simulink model "MotorSpeedController"  (R2016b)
settings: Solver=FixedStepAuto  StartTime=0.0  StopTime=10.0  RelTol=1e-3
PreLoadFcn:
  | waijung.modelPreload; % Required for working with Waijung Blockset. Do not remove.
InitFcn:
  | cubeparameters
undefined symbols (not defined in the file): K, Link, LQFP100, ST, STM32F407VG, STM32F4DISCOVERY, Ts
libraries: stm32f4_io_lib x3, simulink x1, stm32f4_adc_lib x1, stm32f4_device_config_lib x1, BC_USB x1
CloseFcn:
  | waijung.modelClose; % Required for working with Waijung Blockset. Do not remove.
settings Model: Creator=Wall  LastModifiedBy=Wall
settings OptimizationCC: DefaultParameterBehavior=Inlined
settings DebuggingCC: ParameterTunabilityLossMsg=error
settings HardwareCC: ProdBitPerPointer=32  ProdBitPerSizeT=32  ProdBitPerPtrDiffT=32  ProdLargestAtomicFloat=None  ProdIntDivRoundTo=Undefined  ProdWordSize=32  ProdHWDeviceType=ARM Compatible->Cortex - M4  TargetEndianess=LittleEndian  TargetHWDeviceType=ARM Compatible->Cortex - M4
settings RTWCC: SystemTargetFile=stm32f4.tlc  GenerateMakefile=off  TemplateMakefile=ert_default_tmf  Description=STM32F4 Target  GenerateReport=on  IncludeHyperlinkInReport=on  GenerateTraceInfo=on  GenerateTraceReport=on  GenerateTraceReportSl=on  GenerateTraceReportSf=on  GenerateTraceReportEml=on
settings CodeAppCC: ForceParamTrailComments=on  IgnoreCustomStorageClasses=off  OperatorAnnotations=on  SimulinkDataObjDesc=on  SFDataObjDesc=on  MATLABFcnDesc=on  InsertBlockDesc=on  MATLABSourceComments=on
settings STFCustomTargetCC: TargetLangStandard=C99 (ISO)  ModelReferenceCompliant=off  CombineOutputUpdateFcns=on  ERTCustomFileBanners=on  SupportContinuousTime=off  SupportNonInlinedSFcns=off  RemoveResetFunc=on  MATLABClassNameForMDSCustomization=Simulink.SoftwareTarget.ERTCustomization  GRTInterface=off  SystemTargetFile=stm32f4.tlc
settings ERTTargetCC: TargetLangStandard=C99 (ISO)  ModelReferenceCompliant=off  ParMdlRefBuildCompliant=off  CompOptLevelCompliant=off  ConcurrentExecutionCompliant=off  ERTFirstTimeCompliant=off  ModelStepFunctionPrototypeControlCompliant=off  CPPClassGenCompliant=off  UseToolchainInfoCompliant=off  InlinedParameterPlacement=NonHierarchical  ERTSrcFileBannerTemplate=stm32f4_code_template.cgt  ERTHdrFileBannerTemplate=stm32f4_code_template.cgt  ERTDataSrcFileTemplate=stm32f4_code_template.cgt  ERTDataHdrFileTemplate=stm32f4_code_template.cgt  ERTCustomFileTemplate=stm32f4_file_process.tlc

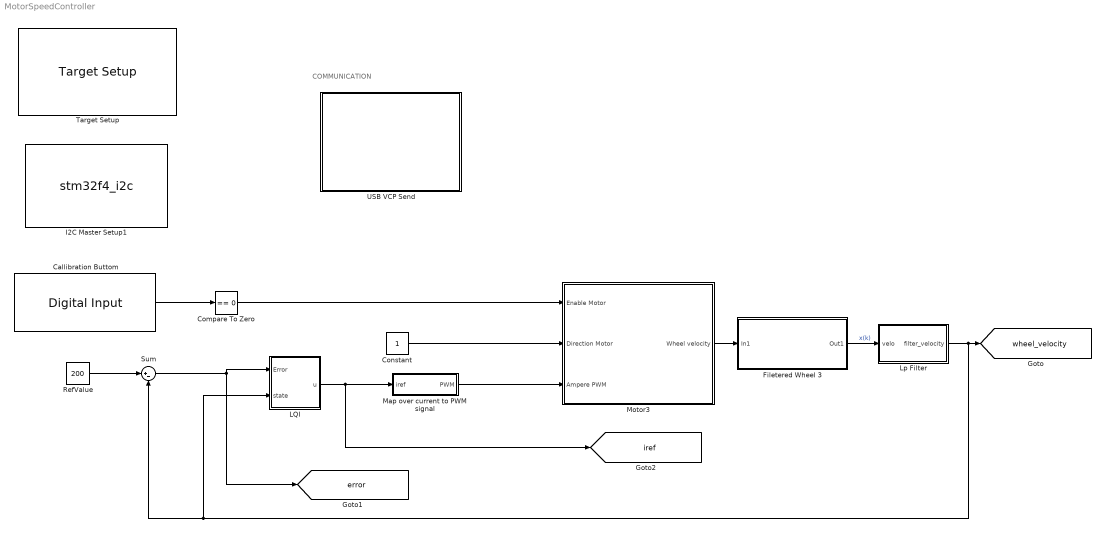
== system MotorSpeedController ==
  note: COMMUNICATION
  Callibration Buttom : stm32f4_io_lib/Digital Input  port=E  speed=100  porttype=Pull Up  porttypestr=UP  use_pin0=off  use_pin1=off  use_pin2=off  use_pin3=off  use_pin4=off  use_pin5=off  use_pin6=off  use_pin7=off  use_pin8=off  use_pin9=off  use_pin10=on  use_pin11=off  use_pin12=off  use_pin13=off  use_pin14=off  use_pin15=off  pinstr=GPIO_Pin_10  usedpinarray="[0  0  0  0  0  0  0  0  0  0  1  0  0  0  0  0]"  bitbandingstr="#define CallibrationButtom_E10 Peripheral_BB(GPIOE->IDR, 10)  /* Output pin */"  sampletime=Ts.controller  sampletimestr=0.016  blockid=CallibrationButtom  enablecustomportlabel=off  glabalinit=off  cinputportlabel=In1, In2  coutputportlabel=Out1, Out2
  Compare To Zero : simulink/Logic and Bit Operations/Compare To Zero  relop===  OutDataTypeStr=boolean
  Constant : Constant  SampleTime=Ts.controller
  Filetered Wheel 3 : Subsystem
  I2C Master Setup1 : S-Function  FunctionName=stm32f4_i2c  Parameters=configuration,module,transfer,clkspeed,timeout,sdapin,sclpin,writecount,readcount,inputtypearray,outputtypearray,confstr,sampletime,sampletimestr,blockid  SFunctionDeploymentMode=off  EnableBusSupport=off  mask(stm32f4_i2c){configuration=Setup, module=1, lastmodule=1, transfer=Blocking, dutycycle=TLow/THigh = 2, clkspeed=400, timeout=25, writecount=0, readcount=0, sdapin=B9, sclpin=B6, waitwritetime=0, inputtypearray=[0], outputtypearray=[0], confstr=["B","9","B","6","1","1","6","0","I2C_DutyCycle_2","0","off"], sampletime=-1, sampletimestr=0.002, blockid=I2CMasterSetup1}
      mask prompts: module "I2C Module"; lastmodule "Last module"; transfer "Transfer mode"; dutycycle "Duty cycle in fast mode"; clkspeed "Clock speed (kHz)"; timeout "Timeout (ms)"; writecount "Bytes write count"; readcount "Bytes read count"; sdapin "SDA pin"; sclpin "SCL pin"; waitwritetime "Wait write time (ms), default is 0"; inputtypearray "Input type array"; outputtypearray "Output type array"; confstr "Configuration string"; sampletime "Sample time (sec)"; sampletimestr "Compiled sample time (sec) in string"
      mask init:
      | stm32f4_i2c_callback('init');
      mask Help: web(fullfile(waijungdocroot,'stm32f4_i2c_setup.htm'), '-browser')
      mask TypeOptions configuration: Setup | Transaction
      mask Callback configuration: stm32f4_i2c_callback('configuration');
      mask TypeOptions module: 1 | 2 | 3
      mask Callback module: stm32f4_i2c_callback('module');
      mask TypeOptions transfer: Blocking | Non-blocking
      mask TypeOptions dutycycle: TLow/THigh = 16/9 | TLow/THigh = 2
      mask Callback dutycycle: stm32f4_i2c_callback('dutycycle');
      mask Callback writecount: stm32f4_i2c_callback('writecount');
      mask Callback readcount: stm32f4_i2c_callback('readcount');
      mask TypeOptions sdapin: - | B7 | B9
      mask Callback sdapin: stm32f4_i2c_callback('sdapin');
      mask TypeOptions sclpin: - | B6 | B8
      mask Callback sclpin: stm32f4_i2c_callback('sclpin');
      mask Callback confstr: stm32f4_i2c_callback('confstr');
      mask Callback sampletime: stm32f4_i2c_callback('sampletime');
      mask Callback sampletimestr: stm32f4_i2c_callback('sampletimestr');
      mask Callback blockid: stm32f4_i2c_callback('blockid');
      mask Display: text(0.5, 0.5, 'Module: I2C1\nClock: 400kHz\nSDA/SCL Pin: B9/B6','ver','middle','hor','center');
  LQI : Subsystem
  Lp Filter : MATLAB Function  TreatAsAtomicUnit=on
  Map over current to PWM signal : Subsystem
  Motor3 : Subsystem
  RefValue : Constant  Value=200  SampleTime=Ts.controller
  Sum : Sum  Inputs=|+-
  Target Setup : stm32f4_device_config_lib/Target Setup  Priority=100  compiler=GNU ARM  previous_compiler=GNU ARM  mcu=STM32F407VG (LQFP100); STM32F4DISCOVERY  mcustr=STM32F407VG  clockconfig=STM32F4DISCOVERY Default (HSEOSC-8MHz/HCLK-168MHz)  system_stm32f4xx_c_path=C:\waijung15_04a\targets\stm32f4_target\stm32f4\utils\STM32F4xx_AN3988_V1.0.1\stm32f4_default\hseosc8mhz  showmemoryconfiguration=off  stacksize=0x400  heapsize=0x200  enableautocompiledownload=on  fullchiperase=off  programmerinterface=ST-Link  editctrlstr=on  compilercontrolstr=$(patsubst %, -I%, .) -mcpu=cortex-m4 -mthumb -mthumb-interwork -mfloat-abi=hard -mfpu=fpv4-sp-d16 -ffast-math -Wall -Wextra -Ofast  assemblercontrolstr=$(patsubst %, -I%, .) -mcpu=cortex-m4 -mthumb -mthumb-interwork -mfloat-abi=hard -mfpu=fpv4-sp-d16 -ffast-math -Wall -Wextra -Ofast -Wa,-amhls=$(<:.s=.lst) -D__STACK_SIZE=$(STACK_SIZE) -D__HEAP_SIZE=$(HEAP_SIZE)  linkercontrolstr=-T$(LD_SCRIPT) -g -Wl,-Map=$(MAP),--cref,--no-warn-mismatch -mcpu=cortex-m4 -mthumb -mthumb-interwork -mfloat-abi=hard -mfpu=fpv4-sp-d16  runafterdownload=on  execprofile=None  profileruart=1  profilerbaud=115200  profilertxpin=Not used  profilerinitstr=0.002,168000000,336000,115200,0  manualsetsampletime=on  sampletime=0.002  blockid=TargetSetup  systickreloadvalue=336000  hseval=8000000  lastprofileruart=1  hclk=168000000  flashorigin=0x8000000  flashlength=1M  ramorigin=0x20000000  ramlength=112k  useextram=off
  USB VCP Send : Subsystem
  tag scope: error=global, iref=global, wheel_velocity=global
  wires:
  Callibration Buttom/1 -> Compare To Zero/1
  Constant/1 -> Motor3/2("Direction Motor ")
  Motor3/1(Wheel velocity) -> Filetered Wheel 3/1(In1)
  Filetered Wheel 3/1(Out1) -> Lp Filter/1(velo)  "x(k)"
  RefValue/1 -> Sum/1
  Sum/1 -> [error], LQI/1(Error)
  LQI/1(u) -> [iref], Map over current to PWM signal/1(iref)
  Compare To Zero/1 -> Motor3/1(Enable Motor)
  Map over current to PWM signal/1(PWM) -> Motor3/3(Ampere PWM)
  Lp Filter/1(filter_velocity) -> LQI/2(state), Sum/2, [wheel_velocity]

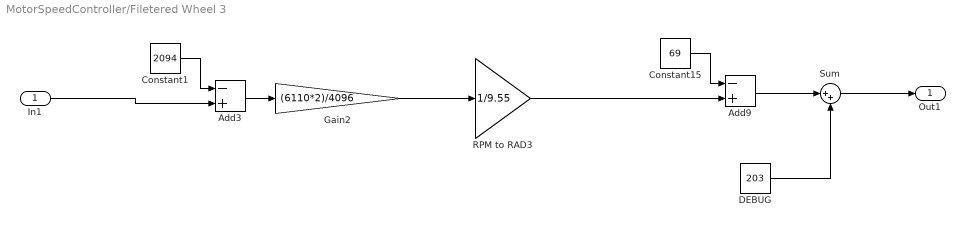
== system MotorSpeedController/Filetered Wheel 3 ==
  In1 : Inport
  Add3 : Sum  Inputs=-+
  Add9 : Sum  Inputs=-+
  Constant1 : Constant  Value=2094  SampleTime=Ts.controller
  Constant15 : Constant  Value=69  SampleTime=Ts.controller
  DEBUG : Constant  Value=203  SampleTime=Ts.controller
  Gain2 : Gain  Gain=(6110*2)/4096
  RPM to RAD3 : Gain  Gain=1/9.55
  Sum : Sum  Inputs=|++
  Out1 : Outport
  wires:
  Gain2/1 -> RPM to RAD3/1
  Add3/1 -> Gain2/1
  Constant1/1 -> Add3/1
  In1/1 -> Add3/2
  Constant15/1 -> Add9/1
  RPM to RAD3/1 -> Add9/2
  Add9/1 -> Sum/1
  Sum/1 -> Out1/1
  DEBUG/1 -> Sum/2

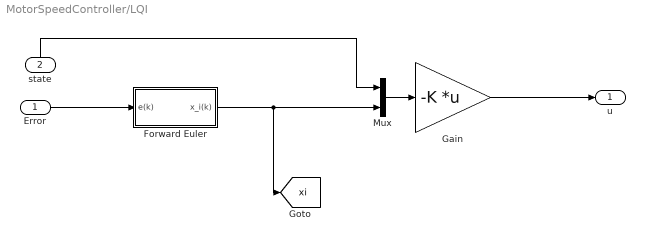
== system MotorSpeedController/LQI ==
  Error : Inport
  state : Inport  Port=2
  Forward Euler : Subsystem
  Gain : Gain  Gain=-K  Multiplication=Matrix(K*u) (u vector)
  Mux : Mux  Inputs=2
  u : Outport
  tag scope: xi=global
  wires:
  Forward Euler/1(x_i(k)) -> [xi], Mux/2
  Mux/1 -> Gain/1
  Error/1 -> Forward Euler/1(e(k))
  state/1 -> Mux/1
  Gain/1 -> u/1

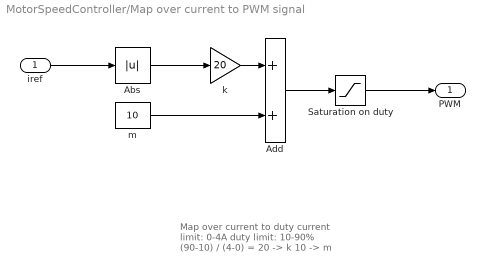
== system MotorSpeedController/Map over current to PWM signal ==
  note: Map over current to duty
      | current limit: 0-4A
      | duty limit: 10-90%
      |
      | (90-10) / (4-0) = 20 -> k
      | 10 -> m
  iref : Inport
  Abs : Abs
  Add : Sum
  Saturation on duty : Saturate  UpperLimit=90  LowerLimit=10  OutDataTypeStr=single
  k : Gain  Gain=20
  m : Constant  Value=10  OutDataTypeStr=single  SampleTime=Ts.controller
  PWM : Outport
  wires:
  Add/1 -> Saturation on duty/1
  Saturation on duty/1 -> PWM/1
  iref/1 -> Abs/1
  Abs/1 -> k/1
  k/1 -> Add/1
  m/1 -> Add/2

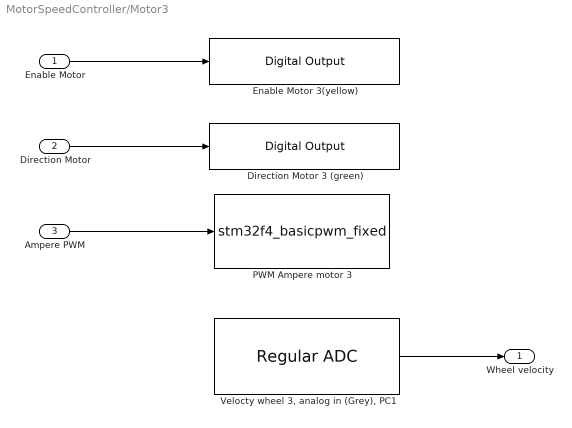
== system MotorSpeedController/Motor3 ==
  Enable Motor : Inport
  "Direction Motor " : Inport  Port=2
  Ampere PWM : Inport  Port=3
  Direction Motor 3 (green) : stm32f4_io_lib/Digital Output  use_bitband=on  port=D  speed=100  porttype=Push Pull  porttypestr=PP  use_pin0=off  use_pin1=off  use_pin2=off  use_pin3=off  use_pin4=off  use_pin5=off  use_pin6=off  use_pin7=off  use_pin8=off  use_pin9=off  use_pin10=off  use_pin11=on  use_pin12=off  use_pin13=off  use_pin14=off  use_pin15=off  pinstr=GPIO_Pin_11  usedpinarray="[0  0  0  0  0  0  0  0  0  0  0  1  0  0  0  0]"  bitbandingstr="#define Motor3DirectionMotor3green_D11 Peripheral_BB(GPIOD->ODR, 11)  /* Output pin */"  sampletime=-1  sampletimestr=0.016  blockid=Motor3DirectionMotor3green  enablecustomportlabel=off  globalinit=off  cinputportlabel=In1, In2  coutputportlabel=0
  Enable Motor 3(yellow) : stm32f4_io_lib/Digital Output  use_bitband=on  port=D  speed=100  porttype=Push Pull  porttypestr=PP  use_pin0=off  use_pin1=off  use_pin2=off  use_pin3=off  use_pin4=off  use_pin5=off  use_pin6=off  use_pin7=off  use_pin8=off  use_pin9=on  use_pin10=off  use_pin11=off  use_pin12=off  use_pin13=off  use_pin14=off  use_pin15=off  pinstr=GPIO_Pin_9  usedpinarray="[0  0  0  0  0  0  0  0  0  1  0  0  0  0  0  0]"  bitbandingstr="#define Motor3EnableMotor3yellow_D9 Peripheral_BB(GPIOD->ODR, 9)  /* Output pin */"  sampletime=-1  sampletimestr=0.016  blockid=Motor3EnableMotor3yellow  enablecustomportlabel=off  globalinit=off  cinputportlabel=In1, In2  coutputportlabel=0
  PWM Ampere motor 3 : S-Function  FunctionName=stm32f4_basicpwm_fixed  Parameters=timer,pwmperiod,uc3m_pwmperiod,ch1pin,ch2pin,ch3pin,ch4pin,sampletime,sampletimestr,blockid,apb,portstr,pinstr,pinmat,timarr,timprescale,chmat,polaritystr  SFunctionDeploymentMode=off  EnableBusSupport=off  mask(stm32f4_basicpwm_fixed){timer=2, pwmperiod=0.02, uc3m_pwmperiod=0.0002, polarity=Active High, polaritystr=TIM_OCPolarity_High, ch1pin=Not available - Do not use, ch2pin=Not available - Do not use, ch3pin=Not available - Do not use, ch4pin=A3, sampletime=-1, sampletimestr=0.016, blockid=Motor3PWMAmperemotor3, portpinstr=,,,A3, enablecustomportlabel=off, cinputportlabel=In1, In2, In3, In4, coutputportlabel=0, callbackgensrccode=off, apb=1, portstr=["A"], pinstr=["GPIO_Pin_3"], pinmat=[1 3], timarr=59999, timprescale=55, chmat=[4]}
      mask prompts: pwmperiod "PWM Period (seconds)"; uc3m_pwmperiod "PWM Signal Period (seconds)"; ch1pin "Channel 1"; ch2pin "Channel 2"; ch3pin "Channel 3"; ch4pin "Channel 4"; sampletime "Sample time (sec)"; sampletimestr "Compiled sample time (sec) in string"; portpinstr "Port pin string"; enablecustomportlabel "Enable custom port labels"; cinputportlabel "Custom input port labels (Ex. In1, In2, In3)"; coutputportlabel "Custom output port labels (Ex. Out1, Out2, Out3)"; callbackgensrccode "Gen source code from callback"; portstr "Port string"; pinstr "Pin string"; pinmat "Pin matrix"; timarr "Timer ARR"; timprescale "Timer PRESCALE"; chmat "Channel order"
      mask help:
      | This block implements basic Edge-aligned Pulse Width Modulation (PWM) generation.
      | All timers are 16-bit. The PWM period is fixed (per timer).
      |
      | This block was fixed by Sr Antonio
      mask init:
      | stm32f4_basicpwm_callback_fixed('init');
      mask Help: web(fullfile(waijungdocroot,'stm32f4_basicpwm.htm'),'-browser')
      mask TypeOptions timer: 1 | 2 | 3 | 4 | 5 | 8 | 9 | 10 | 11 | 12 | 13 | 14
      mask Callback timer: stm32f4_basicpwm_callback_fixed('timer');
      mask Callback pwmperiod: stm32f4_basicpwm_callback_fixed('pwmperiod');
      mask Callback uc3m_pwmperiod: stm32f4_basicpwm_callback_fixed('uc3m_pwmperiod');
      mask TypeOptions polarity: Active High | Active Low
      mask Callback polarity: stm32f4_basicpwm_callback_fixed('polarity');
      mask TypeOptions ch1pin: Not available - Do not use | A0 | A5
      mask Callback ch1pin: stm32f4_basicpwm_callback_fixed('ch1pin');
      mask TypeOptions ch2pin: Not available - Do not use | A1 | B3
      mask Callback ch2pin: stm32f4_basicpwm_callback_fixed('ch2pin');
      mask TypeOptions ch3pin: Not available - Do not use | A2 | B10
      mask Callback ch3pin: stm32f4_basicpwm_callback_fixed('ch3pin');
      mask TypeOptions ch4pin: Not available - Do not use | A3 | B11
      mask Callback ch4pin: stm32f4_basicpwm_callback_fixed('ch4pin');
      mask Callback sampletime: stm32f4_basicpwm_callback_fixed('sampletime');
      mask Callback sampletimestr: stm32f4_basicpwm_callback_fixed('sampletimestr');
      mask Callback blockid: stm32f4_basicpwm_callback_fixed('blockid');
      mask Callback enablecustomportlabel: stm32f4_basicpwm_callback_fixed('enablecustomportlabel')
      mask Display: text(0.95, 0.5, 'UC3M FIXED\nTimer: 2\nPolarity: Active High\nPeriod (sec): 0.0002\nTs (sec): -1','ver','middle','hor','right');port_label('input', 1,'CH4 (A3)')
  "Velocty wheel 3, analog in (Grey), PC1" : stm32f4_adc_lib/Regular ADC  adcmodule=3  outputdatatype=Single  prescaler=2  prescalerstr=ADC_Prescaler_Div2  chsamplingtime=Auto  chsamplingtimestr=ADC_SampleTime_480Cycles  read_an0=off  read_an1=off  read_an2=off  read_an3=off  read_an4=off  read_an5=off  read_an6=off  read_an7=off  read_an8=off  read_an9=off  read_an10=off  read_an11=on  read_an12=off  read_an13=off  read_an14=off  read_an15=off  read_an16=off  read_an17=off  read_an18=off  pinstr=GPIO_Pin_11  usedpinarray="[0  0  0  0  0  0  0  0  0  0  0  1  0  0  0  0  0  0  0]"  usedportidarray=[2]  usedpinidarray=[1]  usedpinidcount=1  sampletime=Ts.controller  blockid=Motor3Veloctywheel3analoginGreyPC1  enablecustomportlabel=off  cinputportlabel=0  coutputportlabel=Out1, Out2
  Wheel velocity : Outport
  wires:
  Ampere PWM/1 -> PWM Ampere motor 3/1
  "Direction Motor "/1 -> Direction Motor 3 (green)/1
  "Velocty wheel 3, analog in (Grey), PC1"/1 -> Wheel velocity/1
  Enable Motor/1 -> Enable Motor 3(yellow)/1

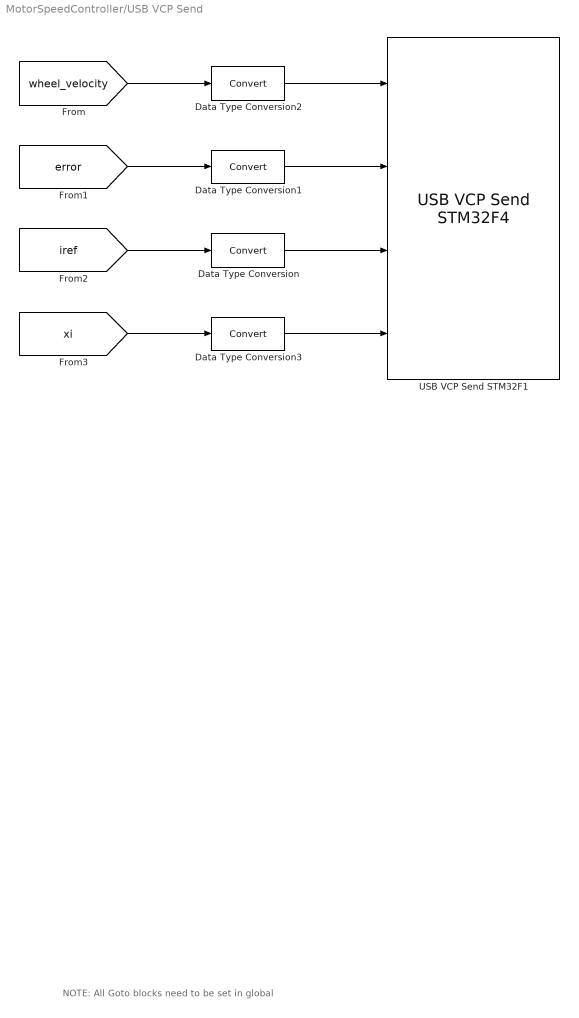
== system MotorSpeedController/USB VCP Send ==
  note: NOTE: All Goto blocks need to be set in global
  Data Type Conversion{,1..3} (4 alike) : DataTypeConversion
  USB VCP Send STM32F1 : BC_USB/USB VCP Send STM32F4  speed="USB 1.1   12Mbit/s"  data_size=2048 Bytes  header_data='0E 0E'  binary_data='single single single single'  terminator_data='0A 0A'  sampletime=Ts.base
  wires:
  [wheel_velocity] -> Data Type Conversion2/1
  [error] -> Data Type Conversion1/1
  [iref] -> Data Type Conversion/1
  Data Type Conversion/1 -> USB VCP Send STM32F1/3
  Data Type Conversion1/1 -> USB VCP Send STM32F1/2
  Data Type Conversion2/1 -> USB VCP Send STM32F1/1
  [xi] -> Data Type Conversion3/1
  Data Type Conversion3/1 -> USB VCP Send STM32F1/4

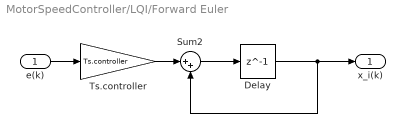
== system MotorSpeedController/LQI/Forward Euler ==
  e(k) : Inport
  Delay : Delay  DelayLength=1
  Sum2 : Sum  Inputs=|++
  Ts.controller : Gain  Gain=Ts.controller
  x_i(k) : Outport
  wires:
  Sum2/1 -> Delay/1
  e(k)/1 -> Ts.controller/1
  Ts.controller/1 -> Sum2/1
  Delay/1 -> Sum2/2, x_i(k)/1

== matlab function MotorSpeedController/Lp Filter ==
  data: velo input; filter_velocity output; Ts parameter
function filter_velocity  = velocity(velo, Ts)

persistent f_velo;
persistent L_velo;


if isempty(f_velo)
   f_velo = 0;
   
   Tf_velo = 4;         % Time Constant % 0.04
   L_velo  = Ts.controller/(Tf_velo + Ts.controller);  % Filter gain
end

% LP Filter
f_velo = (1-L_velo) * f_velo + L_velo * velo;
filter_velocity = f_velo;
